simulink model "SingleIntersection"  (R2017a)
settings: Solver=VariableStepAuto  StartTime=0.0  StopTime=80  RelTol=1e-3
PreLoadFcn:
  | init_func
undefined symbols (not defined in the file or in its folder): m
settings Model: Creator=nebneBgnahZ  LastModifiedBy=nebneBgnahZ

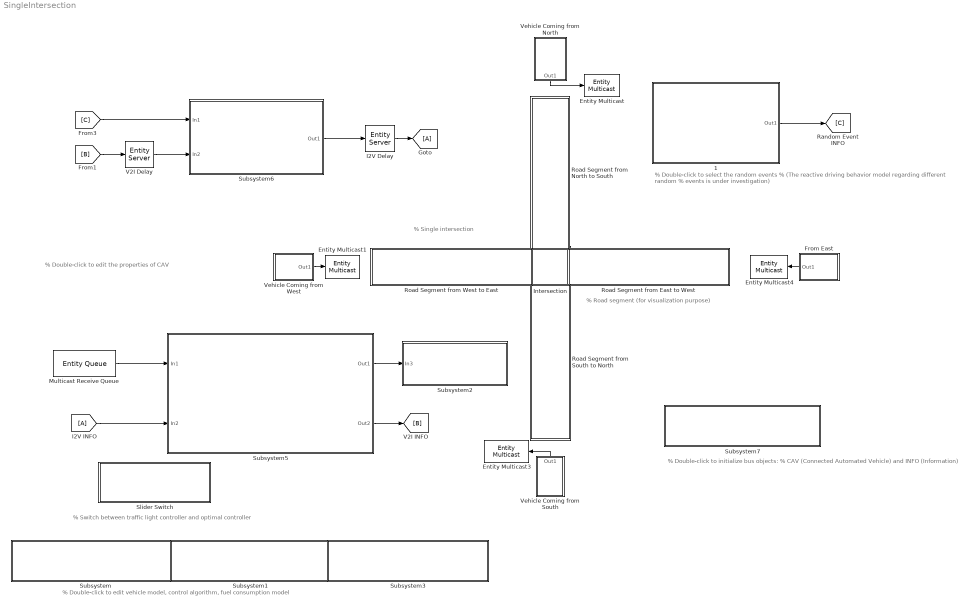
== system SingleIntersection ==
  note: % Switch between traffic light controller and optimal controller
  note: % Double-click to edit vehicle model, control algorithm, fuel consumption model
  note: % Double-click to select the random events
      | % (The reactive driving behavior model regarding different random % events is under investigation)
  note: % Double-click to edit the properties of CAV
  note: % Double-click to initialize bus objects:
      | % CAV (Connected Automated Vehicle) and INFO (Information)
  note: % Single intersection
  note: % Road segment (for visualization purpose)
  " 1" : Subsystem  mask(Random events){Parameter1=Red Light Violation Warning}
      mask help: Random events do not only refer to vehicle arrival, lane change, and turn, but they also include events that may cause safety issues. Generally, all such random events can be categorized into two classes, depending on whether they are caused by vehicles or by the infrastructure/environment.
      mask TypeOptions Parameter1: Red Light Violation Warning | Curve Speed Warning | Stop Sign Gap Assist | Spot Weather Impact Warning | Reduced Speed/ Work Zone Warning | Pedestrian in Signalized Crosswalk Warning (Transit) | Emergency Electronic Brake Lights (EEBL) | Forward Collision Warning (FCW) | Intersection Movement Assist (IMA) | Left Turn Assist (LTA) | Blind Spot/ Lane Change Warning (BSW/LCW) | Do Not Pass Warning (DNPW) | Vehicle Turning Right in Front of Bus Warning (Transit)
      mask Display:
      | %image('figs/environment.jpg');
      | disp('Random Events')
  Entity Multicast{,1,3..4} (4 alike) : EntityMulticast  InputPortMessageModes=m  MulticastTag=CAV
  From East : Subsystem  mask(Connected Automated Vehicles (CAVs)){modelpopup=Basic model, umin=[], umax=[], vmin=[], vmax=[], length=0, cf=0, cr=0, lf=0, lr=0}
      mask prompts: modelpopup "Vehicle Model Selection"; umin "Maximum Deceleration"; umax "Maximum Acceleration"; vmin "Minimum Speed"; vmax "Maximum Speed"; cf "Front Tire Cornering Stiffness"; cr "Rear Tire Cornering Stiffness"; lf "Distance from CoG to Front Axels"; lr "Distance from CoG to Rear Axels"
      mask help: Vehicles, assumed to be CAVs, should possess the ability to communicate with the controller, the coordinator, and other vehicles in the network. CAVs can differ in driver models, for instance, motion dynamics, control mechanism, and fuel consumption dynamics.
      mask TypeOptions modelpopup: Basic model | Kinematic model | Dynamic model | User-defined
      mask Callback modelpopup:
      | % Get the mask parameter values. This is a cell
      | %   array of character vectors.
      | maskStr = get_param(gcb,'modelpopup');
      | 
      | % The pop-up menu is the first mask parameter.
      | %   Check the value selected in the pop-up
      | if strcmp(maskStr(1),'U')
      | 
      | 
      |     % Set the visibility of both parameters on when
      |     %   User-defined is selected in the pop-up.
      | 
      |     set_param(gcb,'MaskVisibilities',{'on';'on';'on';'on';'on';'on';'on';'on';'on';'on';}),
      | 
      | elseif strcmp(maskStr(1),'B')
      | 
      |     % Turn off the visibility of the Value field
      |     %   when User-defined is not selected.
      | 
      |     set_param(gcb,'MaskVisibilities',{'on';'on';'on';'on';'on';'off';'off';'off';'off';'off';}),
      | 
      |     % Set the character vector in the Values field equal to the
      |     % character vector selected in the Gain pop-up menu.
      | 
      |     %maskStr{2}=maskStr{1};
      | 
      | 
      | elseif strcmp(maskStr(1),'K')
      | 
      |     set_param(gcb,'MaskVisibilities',{'on';'on';'on';'on';'on';'on';'off';'off';'off';'off';}),
      | 
      | else
      | 
      |     set_param(gcb,'MaskVisibilities',{'on';'on';'on';'on';'on';'off';'on';'on';'on';'on';}),
      | 
      | end
      mask Display: image('figs/CAV3.png');
  I2V Delay : EntityServer  InputPortMessageModes=m  OutputPortMessageModes=m  Capacity=Inf  ServiceTimeValue=0
  Intersection : Subsystem
      mask Display: image('figs/inter.png');
  Multicast Receive Queue : EntityQueue  OutputPortMessageModes=m  Capacity=100  EntityArrivalSource=Multicast  MulticastTag=CAV
      settings: OutputPortMap=o5
  Road Segment from East to West : Subsystem
      mask Display: image('figs/Roadsegment1.png');
  Road Segment from North to South : Subsystem
      mask Display: image('figs/Roadsegment3.png');
  Road Segment from South to North : Subsystem
      mask Display: image('figs/Roadsegment3.png');
  Road Segment from West to East : Subsystem
      mask Display: image('figs/Roadsegment1.png');
  Slider Switch : Subsystem  DialogController=hmiCreateDDGDialog  IsWebBlock=on  mask(MWDashboardBlock){webBlockId=e7b67206-d875-4afa-ae37-7e6b78c8d41a, webBlockType=sliderswitch, ShowInLibBrowser=on, ShowInitialText=on, HMISrcModelName=SingleIntersection}
      mask prompts: webBlockId "WebBlock Id"; webBlockType "WebBlock Type"; HMISrcModelName "Source Model"
      mask help: SimulinkHMI:dialogs:SwitchDialogDesc
      mask Help: helpview([docroot '/mapfiles/simulink.map'], 'hmi_slider_switch')
      mask Display:
      | if strcmp(get_param(bdroot(gcb),'BlockDiagramType'), 'library')
      |     image([(matlabroot) '/toolbox/simulink/hmi/icons/SliderSwitch.png']);
      | end
  Subsystem : Subsystem
      settings: OpenFcn=edit dynamics.m
      mask Display: disp('Vehicle Motion Dynamics');
  Subsystem1 : Subsystem
      settings: OpenFcn=edit updateAcceleration.m
      mask Display: disp('Vehicle Control Dynamics');
  Subsystem2 : Subsystem
      mask Display: disp('Merging Zone')
  Subsystem3 : Subsystem
      settings: OpenFcn=edit computeFuelConsumption.m
      mask Display: disp('Fuel Consumption Dynamics');
  Subsystem5 : Subsystem
      mask Display:
      | %image('figs/controller.jpg');
      | disp('Control Zone')
  Subsystem6 : Subsystem
      mask Display:
      | %image('figs/coordinator.jpg');
      | disp('Coordinator')
  Subsystem7 : Subsystem
      settings: OpenFcn=init_func
      mask Display: disp('Initialization');
  V2I Delay : EntityServer  InputPortMessageModes=m  OutputPortMessageModes=m  Capacity=Inf  ServiceTimeValue=1
  Vehicle Coming from North : Subsystem  mask(Connected Automated Vehicles (CAVs)){modelpopup=Basic model, umin=[], umax=[], vmin=[], vmax=[], length=0, cf=0, cr=0, lf=0, lr=0}
      mask prompts: modelpopup "Vehicle Model Selection"; umin "Maximum Deceleration"; umax "Maximum Acceleration"; vmin "Minimum Speed"; vmax "Maximum Speed"; cf "Front Tire Cornering Stiffness"; cr "Rear Tire Cornering Stiffness"; lf "Distance from CoG to Front Axels"; lr "Distance from CoG to Rear Axels"
      mask help: Vehicles, assumed to be CAVs, should possess the ability to communicate with the controller, the coordinator, and other vehicles in the network. CAVs can differ in driver models, for instance, motion dynamics, control mechanism, and fuel consumption dynamics.
      mask TypeOptions modelpopup: Basic model | Kinematic model | Dynamic model | User-defined
      mask Callback modelpopup:
      | % Get the mask parameter values. This is a cell
      | %   array of character vectors.
      | maskStr = get_param(gcb,'modelpopup');
      | 
      | % The pop-up menu is the first mask parameter.
      | %   Check the value selected in the pop-up
      | if strcmp(maskStr(1),'U')
      | 
      | 
      |     % Set the visibility of both parameters on when
      |     %   User-defined is selected in the pop-up.
      | 
      |     set_param(gcb,'MaskVisibilities',{'on';'on';'on';'on';'on';'on';'on';'on';'on';'on';}),
      | 
      | elseif strcmp(maskStr(1),'B')
      | 
      |     % Turn off the visibility of the Value field
      |     %   when User-defined is not selected.
      | 
      |     set_param(gcb,'MaskVisibilities',{'on';'on';'on';'on';'on';'off';'off';'off';'off';'off';}),
      | 
      |     % Set the character vector in the Values field equal to the
      |     % character vector selected in the Gain pop-up menu.
      | 
      |     %maskStr{2}=maskStr{1};
      | 
      | 
      | elseif strcmp(maskStr(1),'K')
      | 
      |     set_param(gcb,'MaskVisibilities',{'on';'on';'on';'on';'on';'on';'off';'off';'off';'off';}),
      | 
      | else
      | 
      |     set_param(gcb,'MaskVisibilities',{'on';'on';'on';'on';'on';'off';'on';'on';'on';'on';}),
      | 
      | end
      mask Display: image('figs/CAV4.png');
  Vehicle Coming from South : Subsystem  mask(Connected Automated Vehicles (CAVs)){modelpopup=Basic model, umin=[], umax=[], vmin=[], vmax=[], length=0, cf=0, cr=0, lf=0, lr=0}
      mask prompts: modelpopup "Vehicle Model Selection"; umin "Maximum Deceleration"; umax "Maximum Acceleration"; vmin "Minimum Speed"; vmax "Maximum Speed"; cf "Front Tire Cornering Stiffness"; cr "Rear Tire Cornering Stiffness"; lf "Distance from CoG to Front Axels"; lr "Distance from CoG to Rear Axels"
      mask help: Vehicles, assumed to be CAVs, should possess the ability to communicate with the controller, the coordinator, and other vehicles in the network. CAVs can differ in driver models, for instance, motion dynamics, control mechanism, and fuel consumption dynamics.
      mask TypeOptions modelpopup: Basic model | Kinematic model | Dynamic model | User-defined
      mask Callback modelpopup:
      | % Get the mask parameter values. This is a cell
      | %   array of character vectors.
      | maskStr = get_param(gcb,'modelpopup');
      | 
      | % The pop-up menu is the first mask parameter.
      | %   Check the value selected in the pop-up
      | if strcmp(maskStr(1),'U')
      | 
      | 
      |     % Set the visibility of both parameters on when
      |     %   User-defined is selected in the pop-up.
      | 
      |     set_param(gcb,'MaskVisibilities',{'on';'on';'on';'on';'on';'on';'on';'on';'on';'on';}),
      | 
      | elseif strcmp(maskStr(1),'B')
      | 
      |     % Turn off the visibility of the Value field
      |     %   when User-defined is not selected.
      | 
      |     set_param(gcb,'MaskVisibilities',{'on';'on';'on';'on';'on';'off';'off';'off';'off';'off';}),
      | 
      |     % Set the character vector in the Values field equal to the
      |     % character vector selected in the Gain pop-up menu.
      | 
      |     %maskStr{2}=maskStr{1};
      | 
      | 
      | elseif strcmp(maskStr(1),'K')
      | 
      |     set_param(gcb,'MaskVisibilities',{'on';'on';'on';'on';'on';'on';'off';'off';'off';'off';}),
      | 
      | else
      | 
      |     set_param(gcb,'MaskVisibilities',{'on';'on';'on';'on';'on';'off';'on';'on';'on';'on';}),
      | 
      | end
      mask Display: image('figs/CAV2.png');
  Vehicle Coming from West : Subsystem  mask(Connected Automated Vehicles (CAVs)){modelpopup=Basic model, umin=[], umax=[], vmin=[], vmax=[], length=0, cf=0, cr=0, lf=0, lr=0}
      mask prompts: modelpopup "Vehicle Model Selection"; umin "Maximum Deceleration"; umax "Maximum Acceleration"; vmin "Minimum Speed"; vmax "Maximum Speed"; cf "Front Tire Cornering Stiffness"; cr "Rear Tire Cornering Stiffness"; lf "Distance from CoG to Front Axels"; lr "Distance from CoG to Rear Axels"
      mask help: Vehicles, assumed to be CAVs, should possess the ability to communicate with the controller, the coordinator, and other vehicles in the network. CAVs can differ in driver models, for instance, motion dynamics, control mechanism, and fuel consumption dynamics.
      mask TypeOptions modelpopup: Basic model | Kinematic model | Dynamic model | User-defined
      mask Callback modelpopup:
      | % Get the mask parameter values. This is a cell
      | %   array of character vectors.
      | maskStr = get_param(gcb,'modelpopup');
      | 
      | % The pop-up menu is the first mask parameter.
      | %   Check the value selected in the pop-up
      | if strcmp(maskStr(1),'U')
      | 
      | 
      |     % Set the visibility of both parameters on when
      |     %   User-defined is selected in the pop-up.
      | 
      |     set_param(gcb,'MaskVisibilities',{'on';'on';'on';'on';'on';'on';'on';'on';'on';'on';}),
      | 
      | elseif strcmp(maskStr(1),'B')
      | 
      |     % Turn off the visibility of the Value field
      |     %   when User-defined is not selected.
      | 
      |     set_param(gcb,'MaskVisibilities',{'on';'on';'on';'on';'on';'off';'off';'off';'off';'off';}),
      | 
      |     % Set the character vector in the Values field equal to the
      |     % character vector selected in the Gain pop-up menu.
      | 
      |     %maskStr{2}=maskStr{1};
      | 
      | 
      | elseif strcmp(maskStr(1),'K')
      | 
      |     set_param(gcb,'MaskVisibilities',{'on';'on';'on';'on';'on';'on';'off';'off';'off';'off';}),
      | 
      | else
      | 
      |     set_param(gcb,'MaskVisibilities',{'on';'on';'on';'on';'on';'off';'on';'on';'on';'on';}),
      | 
      | end
      mask Display: image('figs/CAV.png');
  wires:
  Vehicle Coming from South/1(Out1) -> Entity Multicast3/1
  Vehicle Coming from West/1(Out1) -> Entity Multicast1/1
  Vehicle Coming from North/1(Out1) -> Entity Multicast/1
  I2V Delay/1 -> [A]
  [B] -> V2I Delay/1
  " 1"/1(Out1) -> [C]
  Multicast Receive Queue/1 -> Subsystem5/1(In1)
  [A] -> Subsystem5/2(In2)
  Subsystem5/2(Out2) -> [B]
  [C] -> Subsystem6/1(In1)
  V2I Delay/1 -> Subsystem6/2(In2)
  Subsystem6/1(Out1) -> I2V Delay/1
  From East/1(Out1) -> Entity Multicast4/1
  Subsystem5/1(Out1) -> Subsystem2/1(In3)

== system SingleIntersection/ 1 ==
  Random Event : EntityGenerator  OutputPortMessageModes=m  TimeSource=MATLAB action  IntergenerationTimeAction=dt = 1000;  GenerateEntityAtSimulationStart=off  AttributeName=entity  AttributeInitialValue=0  EntityType=Bus object  EntityTypeName=INFO  EntityPriority=100
  Out1 : Outport
  wires:
  Random Event/1 -> Out1/1

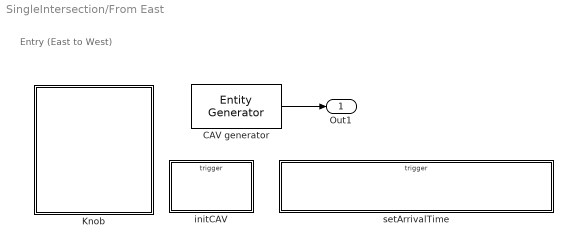
== system SingleIntersection/From East ==
  note: Entry (East to West)
  "CAV generator " : EntityGenerator  DialogController=slde.AttributeBlockDialog  OutputPortMessageModes=m  TimeSource=MATLAB action  IntergenerationTimeAction=|  GenerateEntityAtSimulationStart=off  GenerateAction=|  AttributeName=ID|Speed|ArrivalTime|FinalSpeed|FinalTime|Position|Destination|Lane|Acceleration|coe  AttributeInitialValue=0|1|1|1|1|1|1|1|1|1  EntityType=Bus object  EntityTypeName=CAV
      IntergenerationTimeAction=|
      | mean = 3;
      |  dt = 2.5-mean*log(1-rand());
      | %dt = 1000;
      GenerateAction=|
      | entity.FinalSpeed = 10;
      | [entity.ArrivalTime,...
      |     entity.ID] = setArrivalTime3();
      | entity.Speed = 9 + 3 * rand();
      | entity.Lane = 3;
      | entity.Position = 0;
      | entity.coe = [0, 0, entity.Speed, ...
      |     -entity.Speed * entity.ArrivalTime];
      | dest = [1, 2, 4];
      | idx = ceil(3 * rand()); 
      | entity.Destination = dest(idx);
      | % 0: go straight 1 : right turn 2: left turn
  Knob : Subsystem  DialogController=hmiCreateDDGDialog  IsWebBlock=on  mask(MWDashboardBlock){webBlockId=6ab9dc71-c16a-4f11-9c1c-072b34874571, webBlockType=continuousknob, ShowInLibBrowser=on, ShowInitialText=on, HMISrcModelName=SingleIntersection}
      mask prompts: webBlockId "WebBlock Id"; webBlockType "WebBlock Type"; HMISrcModelName "Source Model"
      mask Help: helpview([docroot '/mapfiles/simulink.map'], 'hmi_knob')
      mask Display:
      | if strcmp(get_param(bdroot(gcb),'BlockDiagramType'), 'library')
      |     image([(matlabroot) '/toolbox/simulink/hmi/icons/ContinuousKnob.png']);
      | end
  initCAV : Subsystem  TreatAsAtomicUnit=on
  setArrivalTime : Subsystem  TreatAsAtomicUnit=on
  Out1 : Outport
  wires:
  "CAV generator "/1 -> Out1/1

== system SingleIntersection/Intersection ==

== system SingleIntersection/Road Segment from East to West ==

== system SingleIntersection/Road Segment from North to South ==

== system SingleIntersection/Road Segment from South to North ==

== system SingleIntersection/Road Segment from West to East ==

== system SingleIntersection/Slider Switch ==

== system SingleIntersection/Subsystem ==

== system SingleIntersection/Subsystem1 ==

== system SingleIntersection/Subsystem2 ==
  In3 : Inport
  Entity Queue : EntityQueue  InputPortMessageModes=m  OutputPortMessageModes=m
      settings: OutputPortMap=o5
  Entity Server : EntityServer  InputPortMessageModes=m  OutputPortMessageModes=m  Capacity=Inf  ServiceTimeSource=MATLAB action  ServiceTimeAction=dt = 30 / entity.FinalSpeed;
  Entity Terminator : EntityTerminator  InputPortMessageModes=m
  wires:
  Entity Queue/1 -> Entity Server/1
  In3/1 -> Entity Queue/1
  Entity Server/1 -> Entity Terminator/1

== system SingleIntersection/Subsystem3 ==

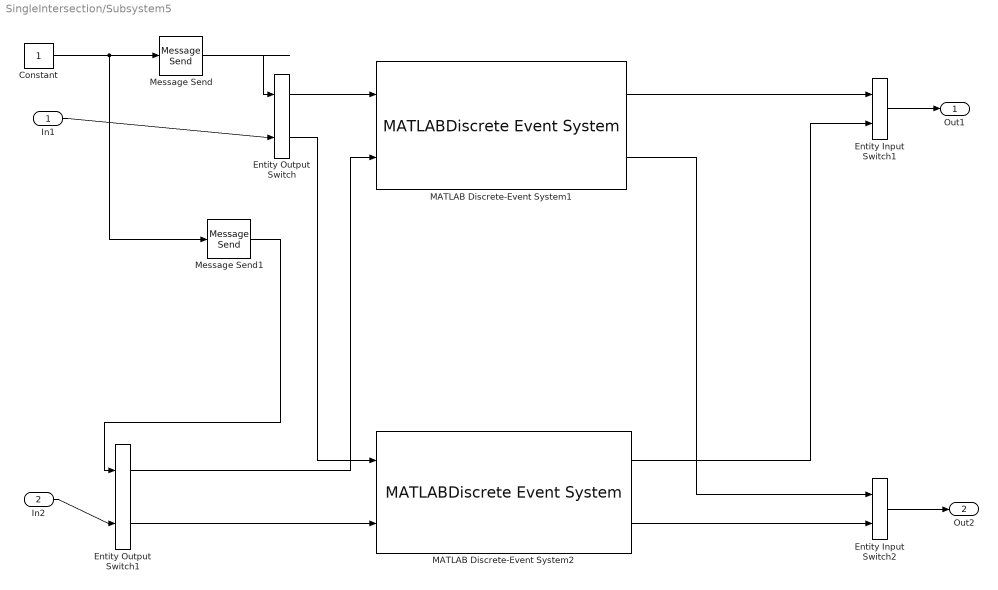
== system SingleIntersection/Subsystem5 ==
  In1 : Inport
  In2 : Inport  Port=2
  Constant : Constant  SampleTime=-1
  Entity Input Switch1 : EntityInputSwitch  InputPortMessageModes=m,m  OutputPortMessageModes=m  SwitchingCriterion=From control port
  Entity Input Switch2 : EntityInputSwitch  InputPortMessageModes=m,m  OutputPortMessageModes=m  SwitchingCriterion=From control port
  Entity Output Switch : EntityOutputSwitch  InputPortMessageModes=m,m  OutputPortMessageModes=m,m  SwitchingCriterion=From control port  SwitchAttributeName=Attribute1
      settings: InputPortMap=u0,u1
  Entity Output Switch1 : EntityOutputSwitch  InputPortMessageModes=m,m  OutputPortMessageModes=m,m  SwitchingCriterion=From control port  SwitchAttributeName=Attribute1
      settings: InputPortMap=u0,u1
  MATLAB Discrete-Event System1 : MATLABDiscreteEventSystem  Description=Coordinator  InputPortMessageModes=m,m  OutputPortMessageModes=m,m  System=Controller  capacity=100  simulation_step=0.01  S=30  L=400  delta=10
      mask Type: Controller
      mask Display:
      | disp('OPTIMAL CONTROLLER');
      | port_label('input',1,'IN');
      | port_label('input',2,'INFO');
      | port_label('output',1,'OUT');
      | port_label('output',2,'INFO');
  MATLAB Discrete-Event System2 : MATLABDiscreteEventSystem  Description=Coordinator  InputPortMessageModes=m,m  OutputPortMessageModes=m,m  System=TrafficLightController  capacity=100  Length=400  simulation_step=0.01  traffic_light_cycle=60  traffic_light_NS=27  traffic_light_NS_yellow=30  traffic_light_EW=57  traffic_light_EW_yellow=60
      mask Type: TrafficLightController
      mask Display:
      | disp('TRAFFIC LIGHT CONTROLLER');
      | port_label('input',1,'IN');
      | port_label('input',2,'INFO');
      | port_label('output',1,'OUT');
      | port_label('output',2,'INFO');
  Message Send : MessageSend  OutputPortMessageModes=m
      settings: InputPortMap=u1
  Message Send1 : MessageSend  OutputPortMessageModes=m
      settings: InputPortMap=u1
  Out1 : Outport
  Out2 : Outport  Port=2
  wires:
  Message Send/1 -> Entity Output Switch/1
  Entity Output Switch1/2 -> MATLAB Discrete-Event System2/2
  Entity Output Switch1/1 -> MATLAB Discrete-Event System1/2
  Entity Output Switch/1 -> MATLAB Discrete-Event System1/1
  MATLAB Discrete-Event System2/1 -> Entity Input Switch1/2
  MATLAB Discrete-Event System2/2 -> Entity Input Switch2/2
  In2/1 -> Entity Output Switch1/2
  Entity Input Switch1/1 -> Out1/1
  Entity Input Switch2/1 -> Out2/1
  Entity Output Switch/2 -> MATLAB Discrete-Event System2/1
  MATLAB Discrete-Event System1/2 -> Entity Input Switch2/1
  In1/1 -> Entity Output Switch/2
  Constant/1 -> Message Send/1, Message Send1/1
  MATLAB Discrete-Event System1/1 -> Entity Input Switch1/1
  Message Send1/1 -> Entity Output Switch1/1

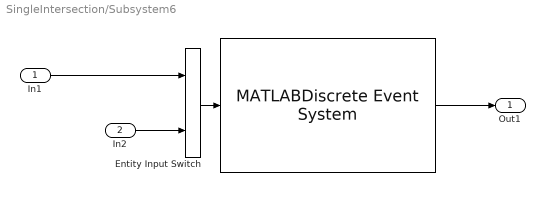
== system SingleIntersection/Subsystem6 ==
  In1 : Inport
  In2 : Inport  Port=2
  " " : MATLABDiscreteEventSystem  InputPortMessageModes=m  OutputPortMessageModes=m  System=Coordinator  capacity=100
      mask Type: Coordinator
      mask Display:
      | disp('COORDINATOR');
      | port_label('input',1,'IN');
      | port_label('output',1,'OUT');
  Entity Input Switch : EntityInputSwitch  InputPortMessageModes=m,m  OutputPortMessageModes=m
  Out1 : Outport
  wires:
  " "/1 -> Out1/1
  In2/1 -> Entity Input Switch/2
  Entity Input Switch/1 -> " "/1
  In1/1 -> Entity Input Switch/1

== system SingleIntersection/Subsystem7 ==

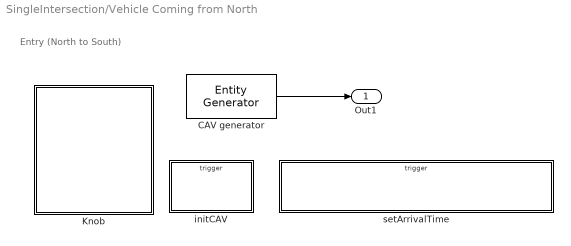
== system SingleIntersection/Vehicle Coming from North ==
  note: Entry (North to South)
  "CAV generator " : EntityGenerator  DialogController=slde.AttributeBlockDialog  OutputPortMessageModes=m  TimeSource=MATLAB action  IntergenerationTimeAction=|  GenerateEntityAtSimulationStart=off  GenerateAction=|  AttributeName=VehicleID|InitialSpeed|ArrivalTime|FinalSpeed|FinalTime|CurrentPosition|Lane|Destination  AttributeInitialValue=0|1|1|1|1|0|1|1  EntityType=Bus object  EntityTypeName=CAV
      IntergenerationTimeAction=|
      | mean = 4;
      |  dt = 1.8-mean*log(1-rand());
      | % dt = 1000;
      GenerateAction=|
      | entity.FinalSpeed = 10;
      | [entity.ArrivalTime,...
      |     entity.ID] = setArrivalTime4();
      | entity.Speed = 8 + 4 * rand();
      | entity.Lane = 4;
      | entity.Position = 0;
      | entity.coe = [0, 0, entity.Speed, ...
      |     -entity.Speed * entity.ArrivalTime];
      | dest = [1, 2, 3];
      | idx = ceil(3 * rand()); 
      | entity.Destination = dest(idx);
  Knob : Subsystem  DialogController=hmiCreateDDGDialog  IsWebBlock=on  mask(MWDashboardBlock){webBlockId=ada4cad8-4919-4fad-b45e-b8882a25ed93, webBlockType=continuousknob, ShowInLibBrowser=on, ShowInitialText=on, HMISrcModelName=SingleIntersection}
      mask prompts: webBlockId "WebBlock Id"; webBlockType "WebBlock Type"; HMISrcModelName "Source Model"
      mask Help: helpview([docroot '/mapfiles/simulink.map'], 'hmi_knob')
      mask Display:
      | if strcmp(get_param(bdroot(gcb),'BlockDiagramType'), 'library')
      |     image([(matlabroot) '/toolbox/simulink/hmi/icons/ContinuousKnob.png']);
      | end
  initCAV : Subsystem  TreatAsAtomicUnit=on
  setArrivalTime : Subsystem  TreatAsAtomicUnit=on
  Out1 : Outport
  wires:
  "CAV generator "/1 -> Out1/1

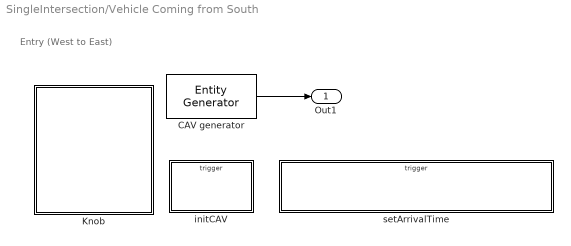
== system SingleIntersection/Vehicle Coming from South ==
  note: Entry (West to East)
  "CAV generator " : EntityGenerator  DialogController=slde.AttributeBlockDialog  OutputPortMessageModes=m  TimeSource=MATLAB action  IntergenerationTimeAction=|  GenerateEntityAtSimulationStart=off  GenerateAction=|  AttributeName=ID|Speed|ArrivalTime|FinalSpeed|FinalTime|Position|Destination|Lane|coe  AttributeInitialValue=0|1|1|1|1|1|1|1|[0 0 0 0]  EntityType=Bus object  EntityTypeName=CAV
      IntergenerationTimeAction=|
      | % dt = 2 * rand();
      | % dt = initCAV2();
      | mean = 2.8;
      | dt = 2.8-mean*log(1-rand());
      | 
      | % dt = 1000;
      GenerateAction=|
      | entity.FinalSpeed = 10;
      | [entity.ArrivalTime,...
      |     entity.ID] = setArrivalTime2();
      | entity.Speed = 9 + 3 * rand();
      | entity.Lane = 2;
      | entity.Position = 0;
      | entity.coe = [0, 0, entity.Speed, ...
      |     -entity.Speed * entity.ArrivalTime];
      | dest = [1, 3, 4];
      | idx = ceil(3 * rand()); 
      | entity.Destination = dest(idx);
      | % 0: go straight 1 : right turn 2: left turn
  Knob : Subsystem  DialogController=hmiCreateDDGDialog  IsWebBlock=on  mask(MWDashboardBlock){webBlockId=f4e2d6bb-37f5-44c7-a610-dc061a88e3e0, webBlockType=continuousknob, ShowInLibBrowser=on, ShowInitialText=on, HMISrcModelName=SingleIntersection}
      mask prompts: webBlockId "WebBlock Id"; webBlockType "WebBlock Type"; HMISrcModelName "Source Model"
      mask Help: helpview([docroot '/mapfiles/simulink.map'], 'hmi_knob')
      mask Display:
      | if strcmp(get_param(bdroot(gcb),'BlockDiagramType'), 'library')
      |     image([(matlabroot) '/toolbox/simulink/hmi/icons/ContinuousKnob.png']);
      | end
  initCAV : Subsystem  TreatAsAtomicUnit=on
  setArrivalTime : Subsystem  TreatAsAtomicUnit=on
  Out1 : Outport
  wires:
  "CAV generator "/1 -> Out1/1

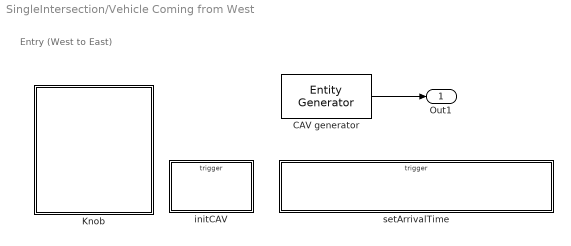
== system SingleIntersection/Vehicle Coming from West ==
  note: Entry (West to East)
  "CAV generator " : EntityGenerator  DialogController=slde.AttributeBlockDialog  OutputPortMessageModes=m  TimeSource=MATLAB action  IntergenerationTimeAction=|  GenerateAction=|  AttributeName=ID|Speed|ArrivalTime|FinalSpeed|FinalTime|Position|Lane|Destination|Acceleration|coe  AttributeInitialValue=0|1|1|1|1|0|1|1|1|[0 0 0 0]  EntityType=Bus object  EntityTypeName=CAV
      IntergenerationTimeAction=|
      | %dt = initCAV();
      | mean = 1.8;
      | dt = 3.8 - mean*log(1-rand());
      GenerateAction=|
      | entity.FinalSpeed = 10;
      | [entity.ArrivalTime,...
      |     entity.ID] = setArrivalTime();
      | %entity.Speed = 8 + 4 * rand();
      | entity.Speed = 12;
      | entity.Lane = 1;
      | entity.Position = 0;
      | entity.coe = [0, 0, entity.Speed,...
      |     - entity.Speed * entity.ArrivalTime];
      | dest = [2, 3, 4];
      | idx = ceil(3 * rand()); 
      | entity.Destination = dest(idx);
      | % 0: go straight 1 : right turn 2: left turn
  Knob : Subsystem  DialogController=hmiCreateDDGDialog  IsWebBlock=on  mask(MWDashboardBlock){webBlockId=60cfeebb-e0ba-4103-a1f5-0e3d9a5610ce, webBlockType=continuousknob, ShowInLibBrowser=on, ShowInitialText=on, HMISrcModelName=SingleIntersection}
      mask prompts: webBlockId "WebBlock Id"; webBlockType "WebBlock Type"; HMISrcModelName "Source Model"
      mask Help: helpview([docroot '/mapfiles/simulink.map'], 'hmi_knob')
      mask Display:
      | if strcmp(get_param(bdroot(gcb),'BlockDiagramType'), 'library')
      |     image([(matlabroot) '/toolbox/simulink/hmi/icons/ContinuousKnob.png']);
      | end
  initCAV : Subsystem  TreatAsAtomicUnit=on
  setArrivalTime : Subsystem  TreatAsAtomicUnit=on
  Out1 : Outport
  wires:
  "CAV generator "/1 -> Out1/1

== system SingleIntersection/From East/Knob ==

== system SingleIntersection/From East/initCAV ==
  initCAV3 : TriggerPort  TriggerType=function-call  IsSimulinkFunction=on  FunctionName=initCAV3  VariantControl=Variant
  "Compute Arrival Time " : Subsystem
  dt : ArgOut  DisableCoverage=on  ArgumentName=dt
  wires:
  "Compute Arrival Time "/1(Out1) -> dt/1

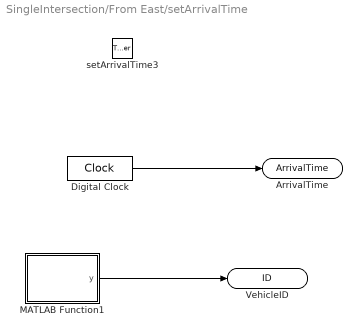
== system SingleIntersection/From East/setArrivalTime ==
  setArrivalTime3 : TriggerPort  TriggerType=function-call  IsSimulinkFunction=on  FunctionName=setArrivalTime3  VariantControl=Variant
  Digital Clock : DigitalClock  SampleTime=-1
  MATLAB Function1 : MATLAB Function  TreatAsAtomicUnit=on
  ArrivalTime : ArgOut  DisableCoverage=on  ArgumentName=ArrivalTime
  VehicleID : ArgOut  DisableCoverage=on  Port=2  ArgumentName=ID
  wires:
  Digital Clock/1 -> ArrivalTime/1
  MATLAB Function1/1(y) -> VehicleID/1

== system SingleIntersection/Vehicle Coming from North/Knob ==

== system SingleIntersection/Vehicle Coming from North/initCAV ==
  initCAV4 : TriggerPort  TriggerType=function-call  IsSimulinkFunction=on  FunctionName=initCAV4  VariantControl=Variant
  "Compute Arrival Time " : Subsystem
  dt : ArgOut  DisableCoverage=on  ArgumentName=dt
  wires:
  "Compute Arrival Time "/1(Out1) -> dt/1

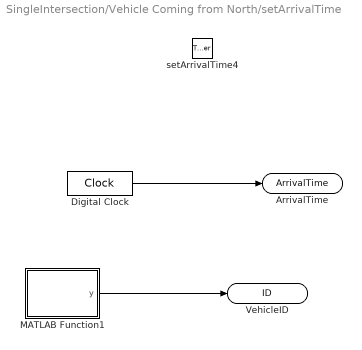
== system SingleIntersection/Vehicle Coming from North/setArrivalTime ==
  setArrivalTime4 : TriggerPort  TriggerType=function-call  IsSimulinkFunction=on  FunctionName=setArrivalTime4  VariantControl=Variant
  Digital Clock : DigitalClock  SampleTime=-1
  MATLAB Function1 : MATLAB Function  TreatAsAtomicUnit=on
  ArrivalTime : ArgOut  DisableCoverage=on  ArgumentName=ArrivalTime
  VehicleID : ArgOut  DisableCoverage=on  Port=2  ArgumentName=ID
  wires:
  Digital Clock/1 -> ArrivalTime/1
  MATLAB Function1/1(y) -> VehicleID/1

== system SingleIntersection/Vehicle Coming from South/Knob ==

== system SingleIntersection/Vehicle Coming from South/initCAV ==
  initCAV : TriggerPort  TriggerType=function-call  IsSimulinkFunction=on  FunctionName=initCAV2  VariantControl=Variant
  "Compute Arrival Time " : Subsystem
  dt : ArgOut  DisableCoverage=on  ArgumentName=dt
  wires:
  "Compute Arrival Time "/1(Out1) -> dt/1

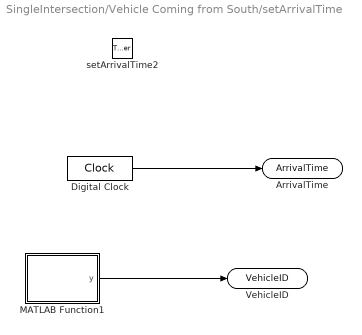
== system SingleIntersection/Vehicle Coming from South/setArrivalTime ==
  setArrivalTime2 : TriggerPort  TriggerType=function-call  IsSimulinkFunction=on  FunctionName=setArrivalTime2  VariantControl=Variant
  Digital Clock : DigitalClock  SampleTime=-1
  MATLAB Function1 : MATLAB Function  TreatAsAtomicUnit=on
  ArrivalTime : ArgOut  DisableCoverage=on  ArgumentName=ArrivalTime
  VehicleID : ArgOut  DisableCoverage=on  Port=2  ArgumentName=VehicleID
  wires:
  Digital Clock/1 -> ArrivalTime/1
  MATLAB Function1/1(y) -> VehicleID/1

== system SingleIntersection/Vehicle Coming from West/Knob ==

== system SingleIntersection/Vehicle Coming from West/initCAV ==
  initCAV : TriggerPort  TriggerType=function-call  IsSimulinkFunction=on  FunctionName=initCAV  VariantControl=Variant
  "Compute Arrival Time " : Subsystem
  dt : ArgOut  DisableCoverage=on  ArgumentName=dt
  wires:
  "Compute Arrival Time "/1(Out1) -> dt/1

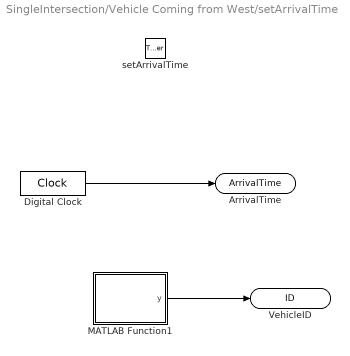
== system SingleIntersection/Vehicle Coming from West/setArrivalTime ==
  setArrivalTime : TriggerPort  TriggerType=function-call  IsSimulinkFunction=on  FunctionName=setArrivalTime  VariantControl=Variant
  Digital Clock : DigitalClock  SampleTime=-1
  MATLAB Function1 : MATLAB Function  TreatAsAtomicUnit=on
  ArrivalTime : ArgOut  DisableCoverage=on  ArgumentName=ArrivalTime
  VehicleID : ArgOut  DisableCoverage=on  Port=2  ArgumentName=ID
  wires:
  Digital Clock/1 -> ArrivalTime/1
  MATLAB Function1/1(y) -> VehicleID/1

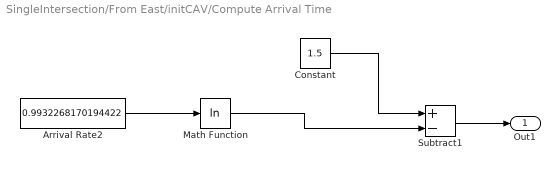
== system SingleIntersection/From East/initCAV/Compute Arrival Time  ==
  "Arrival Rate2 " : Constant  Value=0.9932268170194422  SampleTime=-1
  Constant : Constant  Value=1.5  SampleTime=Inf
  Math Function : Math  Operator=log  SaturateOnIntegerOverflow=on
  Subtract1 : Sum  Inputs=+-
  Out1 : Outport
  wires:
  Subtract1/1 -> Out1/1
  Math Function/1 -> Subtract1/2
  Constant/1 -> Subtract1/1
  "Arrival Rate2 "/1 -> Math Function/1

== system SingleIntersection/Vehicle Coming from North/initCAV/Compute Arrival Time  ==
  "Arrival Rate1 " : Constant  Value=1.006193340207342  SampleTime=-1
  Constant : Constant  Value=2.5  SampleTime=Inf
  Math Function : Math  Operator=log  SaturateOnIntegerOverflow=on
  Subtract1 : Sum  Inputs=+-
  Out1 : Outport
  wires:
  Subtract1/1 -> Out1/1
  Math Function/1 -> Subtract1/2
  Constant/1 -> Subtract1/1
  "Arrival Rate1 "/1 -> Math Function/1

== system SingleIntersection/Vehicle Coming from South/initCAV/Compute Arrival Time  ==
  "Arrival Rate2 " : Constant  Value=0.9932268170194422  SampleTime=-1
  Constant : Constant  Value=1.5  SampleTime=Inf
  Math Function : Math  Operator=log  SaturateOnIntegerOverflow=on
  Subtract1 : Sum  Inputs=+-
  Out1 : Outport
  wires:
  Subtract1/1 -> Out1/1
  Math Function/1 -> Subtract1/2
  Constant/1 -> Subtract1/1
  "Arrival Rate2 "/1 -> Math Function/1

== system SingleIntersection/Vehicle Coming from West/initCAV/Compute Arrival Time  ==
  "Arrival Rate1 " : Constant  Value=1.006193340207342  SampleTime=-1
  Constant : Constant  Value=2  SampleTime=Inf
  Math Function : Math  Operator=log  SaturateOnIntegerOverflow=on
  Subtract1 : Sum  Inputs=+-
  Out1 : Outport
  wires:
  Subtract1/1 -> Out1/1
  Math Function/1 -> Subtract1/2
  Constant/1 -> Subtract1/1
  "Arrival Rate1 "/1 -> Math Function/1

== matlab function SingleIntersection/Vehicle Coming from South/setArrivalTime/MATLAB Function1 ==
  data: y output; FF data_store_memory
function y = getID
global FF

FF = FF + 1;
y = FF;

== matlab function SingleIntersection/Vehicle Coming from West/setArrivalTime/MATLAB Function1 ==
  data: y output; FF data_store_memory
function y = getID()
global FF

FF = FF + 1;
y = FF;

== matlab function SingleIntersection/Vehicle Coming from North/setArrivalTime/MATLAB Function1 ==
  data: y output; FF data_store_memory
function y = getID
global FF

FF = FF + 1;
y = FF;

== matlab function SingleIntersection/From East/setArrivalTime/MATLAB Function1 ==
  data: y output; FF data_store_memory
function y = getID
global FF

FF = FF + 1;
y = FF;
